simulink model "Clutch"  (R2020b)
settings: Solver=VariableStepAuto  StartTime=0.0  StopTime=10.0  RelTol=1e-3
undefined symbols (not defined in the file or in its folder): muk, mus, R
settings Model: Creator=Abhinav dixit  LastModifiedBy=Abhinav dixit

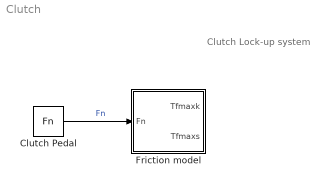
== system Clutch ==
  note: Clutch Lock-up system
  Clutch Pedal : FromWorkspace  VariableName=Fn  ZeroCross=off
  Friction model : Subsystem
  wires:
  Clutch Pedal/1 -> Friction model/1(Fn)  "Fn"

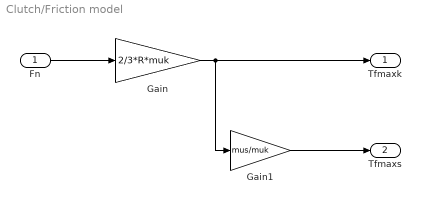
== system Clutch/Friction model ==
  Fn : Inport
  Gain : Gain  Gain=2/3*R*muk
  Gain1 : Gain  Gain=mus/muk
  Tfmaxk : Outport
  Tfmaxs : Outport  Port=2
  wires:
  Gain/1 -> Tfmaxk/1, Gain1/1
  Gain1/1 -> Tfmaxs/1
  Fn/1 -> Gain/1
